simulink model "dtoc"  (Simulink 8.9)
settings: Solver=ode45  StartTime=0.0  StopTime=1  RelTol=1e-3  EnableMultiTasking=on
undefined symbols (not defined in the file): DiscIntNeverNeededParam, Newton, Raphson
libraries: powerlib x9, dspswit3 x6, powerlib_extras x6, simulink_extras x6
settings Model: Creator=Allaudin  LastModifiedBy=hac
settings OptimizationCC: ExpressionDepthLimit=2147483647
settings DebuggingCC: SolverPrmCheckMsg=warning
settings ConfigComp: CovSFcnEnable=off

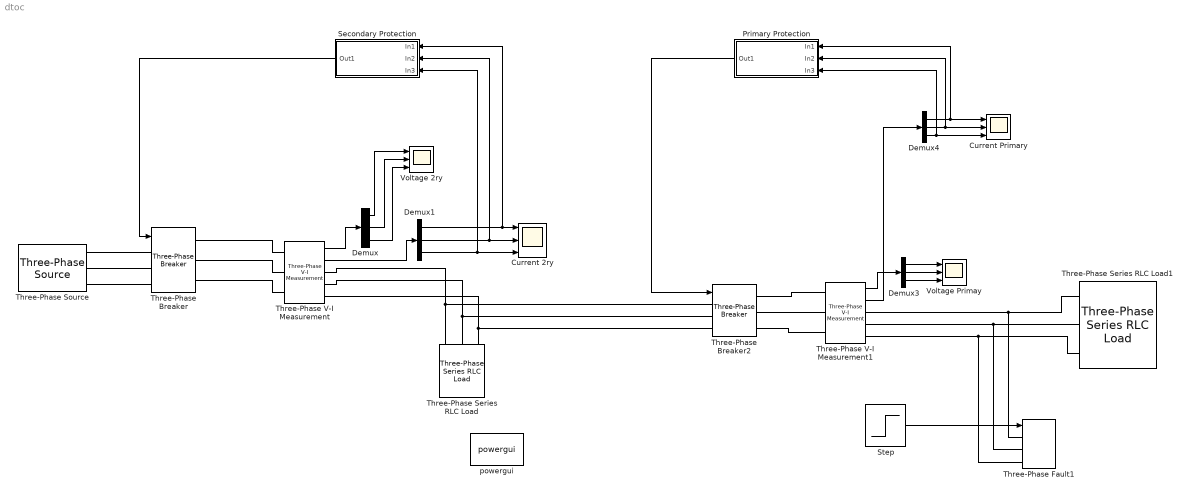
== system dtoc ==
  Current 2ry : Scope  NumInputPorts=3
  Current Primary : Scope  NumInputPorts=3
  Demux{,1,3..4} (4 alike) : Demux  Outputs=3
  Primary Protection : Subsystem
  Secondary Protection : Subsystem
  Step : Step  Time=0.5  SampleTime=0
  Three-Phase Series RLC Load : powerlib/Elements/Three-Phase Series RLC Load  LConnTagsString=A|B|C  Configuration=Y (grounded)  NominalVoltage=11e3  Vabc=[1e3 1e3 1e3]  Vabcp=[1e3 1e3 1e3]  NominalFrequency=50  UnbalancedPower=off  ActivePower=200e6  InductivePower=100  CapacitivePower=0  Pabc=[10e3 9e3 11e3]  QLabc=[100 90 110]  QCabc=[100 90 110]  Pabcp=[10e3 9e3 11e3]  QLabcp=[100 90 110]  QCabcp=[100 90 110]  Measurements=None  LoadType=constant Z
  Three-Phase Series RLC Load1 : powerlib/Elements/Three-Phase Series RLC Load  LConnTagsString=A|B|C  Configuration=Y (grounded)  NominalVoltage=11e3  Vabc=[1e3 1e3 1e3]  Vabcp=[1e3 1e3 1e3]  NominalFrequency=50  UnbalancedPower=off  ActivePower=200e6  InductivePower=100  CapacitivePower=0  Pabc=[10e3 9e3 11e3]  QLabc=[100 90 110]  QCabc=[100 90 110]  Pabcp=[10e3 9e3 11e3]  QLabcp=[100 90 110]  QCabcp=[100 90 110]  Measurements=None  LoadType=constant Z
  Three-Phase V-I Measurement : powerlib/Measurements/Three-Phase V-I Measurement  VoltageMeasurement=phase-to-phase  SetLabelV=off  LabelV=Vabc  Vpu=off  VpuLL=off  CurrentMeasurement=yes  SetLabelI=off  LabelI=Iabc  Ipu=off  Pbase=100e6  Vbase=500e3  OutputType=Complex  PhasorSimulation=off  PSBequivalent=0
  Three-Phase V-I Measurement1 : powerlib/Measurements/Three-Phase V-I Measurement  VoltageMeasurement=phase-to-phase  SetLabelV=off  LabelV=Vabc  Vpu=off  VpuLL=off  CurrentMeasurement=yes  SetLabelI=off  LabelI=Iabc  Ipu=off  Pbase=100e6  Vbase=500e3  OutputType=Complex  PhasorSimulation=off  PSBequivalent=0
  Three-Phase Breaker : powerlib/Elements/Three-Phase Breaker  InitialState=closed  SwitchA=on  SwitchB=on  SwitchC=on  SwitchTimes="[4/60  10/60]"  External=on  BreakerResistance=0.001  SnubberResistance=1e6  SnubberCapacitance=inf  Measurements=None
  Three-Phase Breaker2 : powerlib/Elements/Three-Phase Breaker  InitialState=closed  SwitchA=on  SwitchB=on  SwitchC=on  SwitchTimes="[4/60  10/60]"  External=on  BreakerResistance=0.001  SnubberResistance=1e6  SnubberCapacitance=inf  Measurements=None
  Three-Phase Fault1 : powerlib/Elements/Three-Phase Fault  InitialStates=[0 0 0]  FaultA=on  FaultB=on  FaultC=on  GroundFault=on  SwitchTimes=[ 1/60 5/60]  External=on  SwitchStatus=[1 0]  FaultResistance=0.001  GroundResistance=0.001  SnubberResistance=1e6  SnubberCapacitance=inf  Measurements=None
  Three-Phase Source : powerlib/Electrical Sources/Three-Phase Source  InternalConnection=Yg  VoltagePhases=off  Voltage=11e3  PhaseAngle=0  Voltage_phases=[25e3 25e3 25e3]/sqrt(3)  PhaseAngles_phases=[0 -120 +120]  Frequency=50  NonIdealSource=on  SpecifyImpedance=on  Resistance=0.8929  Inductance=16.58e-3  ShortCircuitLevel=500e6  BaseVoltage=11e3  XRratio=7  BusType=swing  Pref=0  Qref=0  Prefabc=[10e3, 10e3, 10e3]  Qrefabc=[0, 0, 0]  Qmin=-inf  Qmax=inf
  Voltage 2ry : Scope  NumInputPorts=3
  Voltage Primay : Scope  NumInputPorts=3
  powergui : powerlib/powergui  Priority=1  SimulationMode=Discrete  SampleTime=1e-4  frequency=60  Iterations=50  frequencyindice=0  Pbase=100e6  ErrMax=1e-4  UnitsV=kV  UnitsW=MW  buscounter=0  FunctionMessages=off  echomessages=off  EnableUseOfTLC=off  CurrentSourceSwitches=off  DisableSnubberDevices=off  DisableRonSwitches=off  DisableVfSwitches=off  DisplayEquations=off  SolverType=Tustin  Interpol=off  ExternalGateDelay=off  methode=off  Ts=0  x0status=blocks  SPID=off  SwTol=0  HookPort=off  RestoreLinks=warning  ResistiveCurrentMeasurement=off  Frange=[0:2:500]  Ylog=off  Xlog=on  ShowGrid=off  save=off  variable=ZData  structure=0  ZoomFFT=on  StartTime=0.0  cycles=1  DisplayStyle=1  fundamental=60  FreqAxis=off  MaxFrequency=1000  frequencyindicesteady=1  RmsSteady=1  display=off
  wires:
  Three-Phase V-I Measurement/2 -> Demux1/1
  Three-Phase V-I Measurement/1 -> Demux/1
  Demux/1 -> Voltage 2ry/1
  Demux/2 -> Voltage 2ry/2
  Demux/3 -> Voltage 2ry/3
  Demux1/1 -> Secondary Protection/1(In1), Current 2ry/1
  Demux1/2 -> Secondary Protection/2(In2), Current 2ry/2
  Demux1/3 -> Secondary Protection/3(In3), Current 2ry/3
  Demux3/3 -> Voltage Primay/3
  Demux3/2 -> Voltage Primay/2
  Demux3/1 -> Voltage Primay/1
  Three-Phase V-I Measurement1/1 -> Demux3/1
  Demux4/3 -> Primary Protection/3(In3), Current Primary/3
  Demux4/2 -> Primary Protection/2(In2), Current Primary/2
  Demux4/1 -> Primary Protection/1(In1), Current Primary/1
  Three-Phase V-I Measurement1/2 -> Demux4/1
  Secondary Protection/1(Out1) -> Three-Phase Breaker/1
  Step/1 -> Three-Phase Fault1/1
  Primary Protection/1(Out1) -> Three-Phase Breaker2/1
  connections:
  Three-Phase Source/RConn1 -- Three-Phase Breaker/LConn1
  Three-Phase Source/RConn2 -- Three-Phase Breaker/LConn2
  Three-Phase Source/RConn3 -- Three-Phase Breaker/LConn3
  Three-Phase Breaker/RConn1 -- Three-Phase V-I Measurement/LConn1
  Three-Phase Breaker/RConn2 -- Three-Phase V-I Measurement/LConn2
  Three-Phase Breaker/RConn3 -- Three-Phase V-I Measurement/LConn3
  Three-Phase V-I Measurement/RConn2 -- Three-Phase Series RLC Load/LConn2 -- Three-Phase Breaker2/LConn2
  Three-Phase V-I Measurement/RConn3 -- Three-Phase Series RLC Load/LConn3 -- Three-Phase Breaker2/LConn3
  Three-Phase V-I Measurement/RConn1 -- Three-Phase Series RLC Load/LConn1 -- Three-Phase Breaker2/LConn1
  Three-Phase Breaker2/RConn3 -- Three-Phase V-I Measurement1/LConn3
  Three-Phase Breaker2/RConn2 -- Three-Phase V-I Measurement1/LConn2
  Three-Phase Breaker2/RConn1 -- Three-Phase V-I Measurement1/LConn1
  Three-Phase V-I Measurement1/RConn3 -- Three-Phase Fault1/LConn3 -- Three-Phase Series RLC Load1/LConn3
  Three-Phase V-I Measurement1/RConn2 -- Three-Phase Fault1/LConn2 -- Three-Phase Series RLC Load1/LConn2
  Three-Phase V-I Measurement1/RConn1 -- Three-Phase Fault1/LConn1 -- Three-Phase Series RLC Load1/LConn1

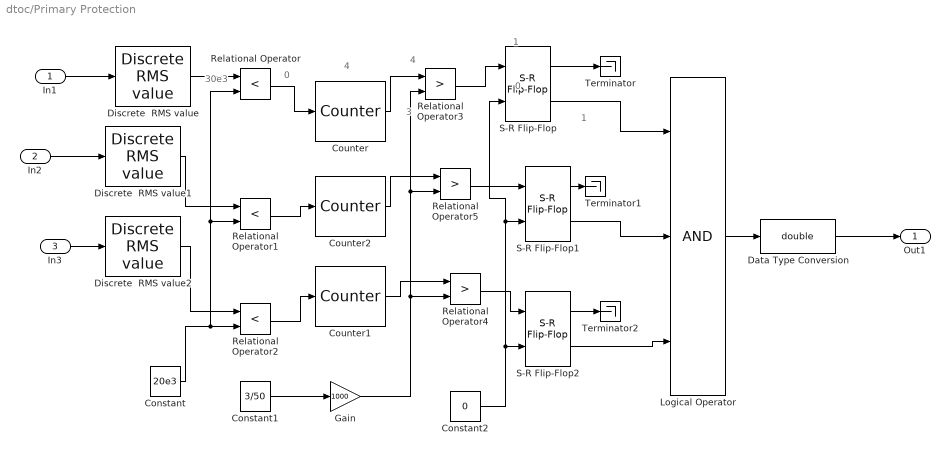
== system dtoc/Primary Protection ==
  note: 0
  note: 30e3
  note: 1
  note: 0
  note: 1
  note: 3
  note: 4
  note: 4
  In1 : Inport
  In2 : Inport  Port=2
  In3 : Inport  Port=3
  Constant : Constant  Value=20e3  OutDataTypeStr=double
  Constant1 : Constant  Value=3/50
  Constant2 : Constant  Value=0  OutDataTypeStr=boolean
  Counter : dspswit3/Counter  Direction=Up  CountEvent=Free running  CounterSize=User defined  MaxCount=1e6  InitialCount=0  Output=Count  HitValue=32  ResetInput=on  SamplesPerFrame=1  Ts=0.001  CntDtype=double  HitDtype=Logical
  Counter1 : dspswit3/Counter  Direction=Up  CountEvent=Free running  CounterSize=User defined  MaxCount=1e6  InitialCount=0  Output=Count  HitValue=32  ResetInput=on  SamplesPerFrame=1  Ts=0.001  CntDtype=double  HitDtype=Logical
  Counter2 : dspswit3/Counter  Direction=Up  CountEvent=Free running  CounterSize=User defined  MaxCount=1e6  InitialCount=0  Output=Count  HitValue=32  ResetInput=on  SamplesPerFrame=1  Ts=0.001  CntDtype=double  HitDtype=Logical
  Data Type Conversion : DataTypeConversion  OutDataTypeStr=double
  Discrete  RMS value : powerlib_extras/Discrete Measurements/Discrete  RMS value  Freq=50  Mag_Init=0  Ts=0.001
  Discrete  RMS value1 : powerlib_extras/Discrete Measurements/Discrete  RMS value  Freq=50  Mag_Init=0  Ts=0.001
  Discrete  RMS value2 : powerlib_extras/Discrete Measurements/Discrete  RMS value  Freq=50  Mag_Init=0  Ts=0.001
  Gain : Gain  Gain=1000  ParamDataTypeStr=double
  Logical Operator : Logic  Inputs=3  AllPortsSameDT=off  OutDataTypeStr=boolean
  Relational Operator : RelationalOperator  Operator=<  OutDataTypeStr=boolean  RndMeth=Nearest
  Relational Operator1 : RelationalOperator  Operator=<  OutDataTypeStr=boolean  RndMeth=Nearest
  Relational Operator2 : RelationalOperator  Operator=<  OutDataTypeStr=boolean  RndMeth=Nearest
  Relational Operator3 : RelationalOperator  Operator=>  OutDataTypeStr=boolean  RndMeth=Nearest
  Relational Operator4 : RelationalOperator  Operator=>  OutDataTypeStr=boolean  RndMeth=Nearest
  Relational Operator5 : RelationalOperator  Operator=>  OutDataTypeStr=boolean  RndMeth=Nearest
  S-R Flip-Flop : simulink_extras/Flip Flops/S-R Flip-Flop  initial_condition=0
  S-R Flip-Flop1 : simulink_extras/Flip Flops/S-R Flip-Flop  initial_condition=0
  S-R Flip-Flop2 : simulink_extras/Flip Flops/S-R Flip-Flop  initial_condition=0
  Terminator : Terminator
  Terminator1 : Terminator
  Terminator2 : Terminator
  Out1 : Outport
  wires:
  In1/1 -> Discrete  RMS value/1
  In2/1 -> Discrete  RMS value1/1
  In3/1 -> Discrete  RMS value2/1
  Constant/1 -> Relational Operator/2, Relational Operator1/2, Relational Operator2/2
  Relational Operator/1 -> Counter/1
  Relational Operator1/1 -> Counter2/1
  Relational Operator2/1 -> Counter1/1
  Constant2/1 -> S-R Flip-Flop/2, S-R Flip-Flop1/2, S-R Flip-Flop2/2
  Logical Operator/1 -> Data Type Conversion/1
  Data Type Conversion/1 -> Out1/1
  Discrete  RMS value/1 -> Relational Operator/1
  Discrete  RMS value1/1 -> Relational Operator1/1
  Discrete  RMS value2/1 -> Relational Operator2/1
  Counter1/1 -> Relational Operator4/1
  Counter2/1 -> Relational Operator5/1
  Counter/1 -> Relational Operator3/1
  Relational Operator4/1 -> S-R Flip-Flop2/1
  Relational Operator5/1 -> S-R Flip-Flop1/1
  Relational Operator3/1 -> S-R Flip-Flop/1
  Constant1/1 -> Gain/1
  Gain/1 -> Relational Operator3/2, Relational Operator5/2, Relational Operator4/2
  S-R Flip-Flop2/2 -> Logical Operator/3
  S-R Flip-Flop2/1 -> Terminator2/1
  S-R Flip-Flop1/2 -> Logical Operator/2
  S-R Flip-Flop1/1 -> Terminator1/1
  S-R Flip-Flop/2 -> Logical Operator/1
  S-R Flip-Flop/1 -> Terminator/1

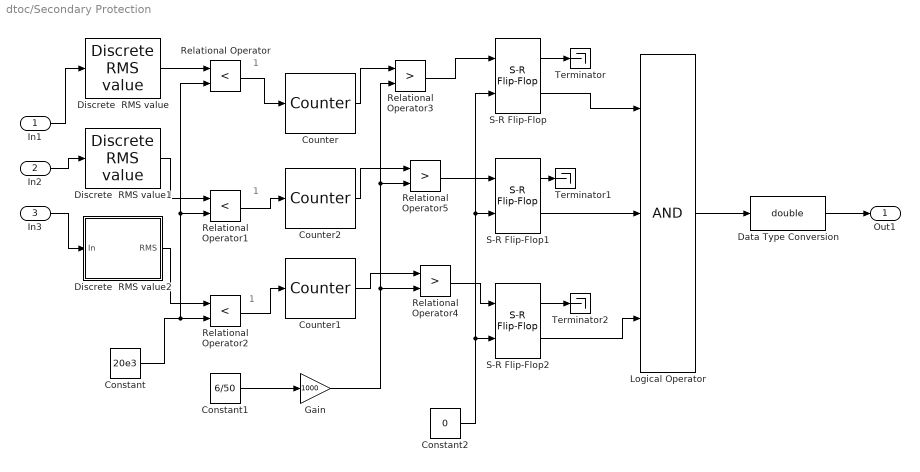
== system dtoc/Secondary Protection ==
  note: 1
  note: 1
  note: 1
  In1 : Inport
  In2 : Inport  Port=2
  In3 : Inport  Port=3
  Constant : Constant  Value=20e3  OutDataTypeStr=double
  Constant1 : Constant  Value=6/50
  Constant2 : Constant  Value=0  OutDataTypeStr=boolean
  Counter : dspswit3/Counter  Direction=Up  CountEvent=Free running  CounterSize=User defined  MaxCount=1e6  InitialCount=0  Output=Count  HitValue=32  ResetInput=on  SamplesPerFrame=1  Ts=0.001  CntDtype=double  HitDtype=Logical
  Counter1 : dspswit3/Counter  Direction=Up  CountEvent=Free running  CounterSize=User defined  MaxCount=1e6  InitialCount=0  Output=Count  HitValue=32  ResetInput=on  SamplesPerFrame=1  Ts=0.001  CntDtype=double  HitDtype=Logical
  Counter2 : dspswit3/Counter  Direction=Up  CountEvent=Free running  CounterSize=User defined  MaxCount=1e6  InitialCount=0  Output=Count  HitValue=32  ResetInput=on  SamplesPerFrame=1  Ts=0.001  CntDtype=double  HitDtype=Logical
  Data Type Conversion : DataTypeConversion  OutDataTypeStr=double
  Discrete  RMS value : powerlib_extras/Discrete Measurements/Discrete  RMS value  Freq=50  Mag_Init=0  Ts=0.001
  Discrete  RMS value1 : powerlib_extras/Discrete Measurements/Discrete  RMS value  Freq=50  Mag_Init=0  Ts=0.001
  Discrete  RMS value2 : Subsystem  AncestorBlock=|  DialogController=POWERSYS.PowerSysDialog  mask(Discrete RMS value){Freq=50, Mag_Init=0, Ts=0.001}
      | powerlib_extras/Discrete
      | Measurements/Discrete 
      | RMS value
      mask prompts: Freq "Fundamental frequency (Hz):"; Mag_Init "Initial magnitude of input:"; Ts "Sample time:"
      mask help:
      | Measure the true root mean square (RMS) value of a signal.
      |
      | NOTE:
      | The Measurements sub-library of the Control and Measurements library contains an improved version of this block.
      mask init:
      | power_initmask();
      mask Help: Please refer to the help of RMS block of the new Control and Measurements library (powerlib_meascontrol) of Simscape Power Systems (Specialized Technology).
      mask Display: disp('RMS\n(discrete)')
  Gain : Gain  Gain=1000  ParamDataTypeStr=double
  Logical Operator : Logic  Inputs=3  AllPortsSameDT=off  OutDataTypeStr=boolean
  Relational Operator : RelationalOperator  Operator=<  OutDataTypeStr=boolean  RndMeth=Nearest
  Relational Operator1 : RelationalOperator  Operator=<  OutDataTypeStr=boolean  RndMeth=Nearest
  Relational Operator2 : RelationalOperator  Operator=<  OutDataTypeStr=boolean  RndMeth=Nearest
  Relational Operator3 : RelationalOperator  Operator=>  OutDataTypeStr=boolean  RndMeth=Nearest
  Relational Operator4 : RelationalOperator  Operator=>  OutDataTypeStr=boolean  RndMeth=Nearest
  Relational Operator5 : RelationalOperator  Operator=>  OutDataTypeStr=boolean  RndMeth=Nearest
  S-R Flip-Flop : simulink_extras/Flip Flops/S-R Flip-Flop  initial_condition=0
  S-R Flip-Flop1 : simulink_extras/Flip Flops/S-R Flip-Flop  initial_condition=0
  S-R Flip-Flop2 : simulink_extras/Flip Flops/S-R Flip-Flop  initial_condition=0
  Terminator : Terminator
  Terminator1 : Terminator
  Terminator2 : Terminator
  Out1 : Outport
  wires:
  In1/1 -> Discrete  RMS value/1
  In2/1 -> Discrete  RMS value1/1
  In3/1 -> Discrete  RMS value2/1(In)
  Constant/1 -> Relational Operator/2, Relational Operator1/2, Relational Operator2/2
  Relational Operator/1 -> Counter/1
  Relational Operator1/1 -> Counter2/1
  Relational Operator2/1 -> Counter1/1
  Constant2/1 -> S-R Flip-Flop/2, S-R Flip-Flop1/2, S-R Flip-Flop2/2
  Logical Operator/1 -> Data Type Conversion/1
  Data Type Conversion/1 -> Out1/1
  Discrete  RMS value/1 -> Relational Operator/1
  Discrete  RMS value1/1 -> Relational Operator1/1
  Discrete  RMS value2/1(RMS) -> Relational Operator2/1
  Counter1/1 -> Relational Operator4/1
  Counter2/1 -> Relational Operator5/1
  Counter/1 -> Relational Operator3/1
  Relational Operator4/1 -> S-R Flip-Flop2/1
  Relational Operator5/1 -> S-R Flip-Flop1/1
  Relational Operator3/1 -> S-R Flip-Flop/1
  Constant1/1 -> Gain/1
  Gain/1 -> Relational Operator3/2, Relational Operator5/2, Relational Operator4/2
  S-R Flip-Flop2/2 -> Logical Operator/3
  S-R Flip-Flop2/1 -> Terminator2/1
  S-R Flip-Flop1/2 -> Logical Operator/2
  S-R Flip-Flop1/1 -> Terminator1/1
  S-R Flip-Flop/2 -> Logical Operator/1
  S-R Flip-Flop/1 -> Terminator/1

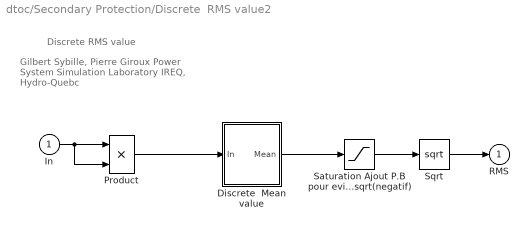
== system dtoc/Secondary Protection/Discrete  RMS value2 ==
  note: Discrete RMS value
  note: Gilbert Sybille, Pierre Giroux
      | Power System Simulation Laboratory
      | IREQ, Hydro-Quebc
  In : Inport
  Discrete  Mean value : Subsystem  AncestorBlock=|  DialogController=POWERSYS.PowerSysDialog  mask(Discrete Mean value){Freq=Freq, Vinit=Mag_Init*Mag_Init, Ts=Ts}
      | powerlib_extras/Discrete
      | Measurements/Discrete 
      | Mean value
      mask prompts: Freq "Fundamental frequency (Hz):"; Vinit "Initial input (DC component):"; Ts "Sample time:"
      mask help:
      | Compute the mean value of the input signal over a running window of one cycle of the specified fundamental frequency. For the first cycle of simulation, the output is held constant to the specified initial input value.
      |
      | NOTE:
      | The Measurements sub-library of the Control and Measurements library contains an improved version of this block.
      mask init:
      | SamplesPerCycle=1/Freq/Ts;
      | RoundSamplesPerCycle=ceil(SamplesPerCycle);
      | Delay=RoundSamplesPerCycle*Ts;
      | Corr1=(SamplesPerCycle-RoundSamplesPerCycle)/2;
      | Corr2=(SamplesPerCycle-RoundSamplesPerCycle)/SamplesPerCycle;
      | K1=Corr1*Corr2;
      | K2=Corr2 + Corr1*Corr2;
      | power_initmask();
      mask Help: This block is part of a subset of blocks in the Extras library that does not have documentation associated with it, other than the block mask description.
      mask Display: disp('Mean\n(discrete)')
  Product : Product  SaturateOnIntegerOverflow=on  InputSameDT=on  OutDataTypeStr=Inherit: Same as first input
  Saturation Ajout P.B pour eviter  sqrt(negatif) : Saturate  UpperLimit=Inf  LowerLimit=0
  Sqrt : Sqrt  AlgorithmType=Newton-Raphson  SaturateOnIntegerOverflow=on
  RMS : Outport  InitialOutput=0
  wires:
  Saturation Ajout P.B pour eviter  sqrt(negatif)/1 -> Sqrt/1
  Discrete  Mean value/1(Mean) -> Saturation Ajout P.B pour eviter  sqrt(negatif)/1
  Product/1 -> Discrete  Mean value/1(In)
  Sqrt/1 -> RMS/1
  In/1 -> Product/1, Product/2

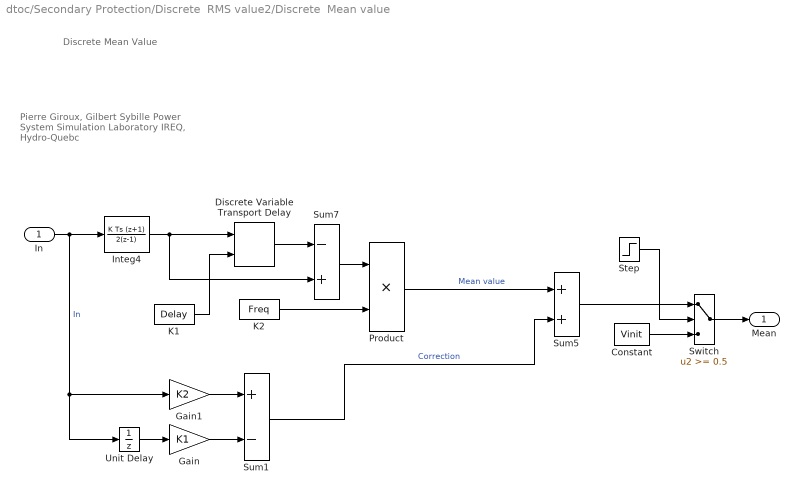
== system dtoc/Secondary Protection/Discrete  RMS value2/Discrete  Mean value ==
  note: Pierre Giroux, Gilbert Sybille
      | Power System Simulation Laboratory
      | IREQ, Hydro-Quebc
  note: Discrete Mean Value
  In : Inport
  Constant : Constant  Value=Vinit  SampleTime=Ts
  Discrete Variable Transport Delay : powerlib_extras/Discrete  Control Blocks/Discrete Variable Transport Delay  MaxDelay=Delay+Ts  InitialValue=0  Ts=Ts
  Gain : Gain  Gain=K1  SaturateOnIntegerOverflow=on  OutDataTypeStr=Inherit: Same as input  ParamDataTypeStr=Inherit: Same as input
  Gain1 : Gain  Gain=K2  SaturateOnIntegerOverflow=on  OutDataTypeStr=Inherit: Same as input  ParamDataTypeStr=Inherit: Same as input
  Integ4 : DiscreteIntegrator  IntegratorMethod=Integration: Trapezoidal  SampleTime=Ts  ICPrevOutput=DiscIntNeverNeededParam  ICPrevScaledInput=DiscIntNeverNeededParam
  K1 : Constant  Value=Delay  SampleTime=Ts
  K2 : Constant  Value=Freq  SampleTime=Ts
  Product : Product  SaturateOnIntegerOverflow=on  InputSameDT=on  OutDataTypeStr=Inherit: Same as first input
  Step : Step  Time=1/Freq  SampleTime=Ts
  Sum1 : Sum  Inputs=+-  SaturateOnIntegerOverflow=on  InputSameDT=on  OutDataTypeStr=Inherit: Same as first input
  Sum5 : Sum  SaturateOnIntegerOverflow=on  InputSameDT=on  OutDataTypeStr=Inherit: Same as first input
  Sum7 : Sum  Inputs=-+  SaturateOnIntegerOverflow=on  InputSameDT=on  OutDataTypeStr=Inherit: Same as first input
  Switch : Switch  Threshold=0.5  InputSameDT=on
  Unit Delay : UnitDelay  SampleTime=Ts
  Mean : Outport
  wires:
  Product/1 -> Sum5/1  "Mean value"
  Sum7/1 -> Product/1
  Integ4/1 -> Discrete Variable Transport Delay/1, Sum7/2
  K2/1 -> Product/2
  In/1 -> Integ4/1, Gain1/1, Unit Delay/1  "In"
  Sum5/1 -> Switch/1
  Step/1 -> Switch/2
  Constant/1 -> Switch/3
  Switch/1 -> Mean/1
  Discrete Variable Transport Delay/1 -> Sum7/1
  K1/1 -> Discrete Variable Transport Delay/2
  Gain1/1 -> Sum1/1
  Unit Delay/1 -> Gain/1
  Gain/1 -> Sum1/2
  Sum1/1 -> Sum5/2  "Correction"
